simulink library "gmt_Simulink_R2023a"  (R2023a)
settings: Solver=VariableStepAuto  StartTime=0.0  StopTime=10.0  RelTol=1e-3
undefined symbols (not defined in the file or in its folder): MainTank
settings Model: Creator=caksland  LastModifiedBy=jmp8430
settings OptimizationCC: ReuseModelBlockBuffer=off
settings ConfigComp: CovBoundaryAbsTol=1.0e-5

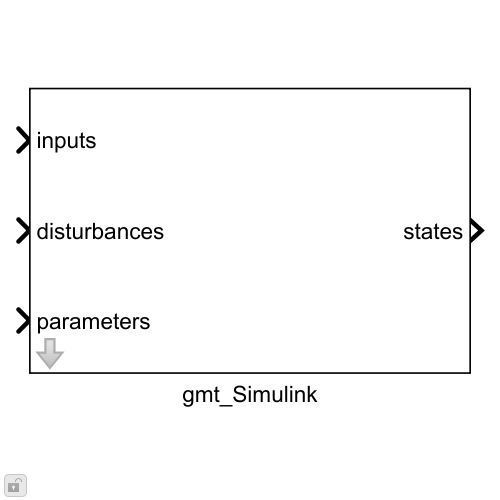
[thumbnail: Simulink's stored preview of the top-level diagram]
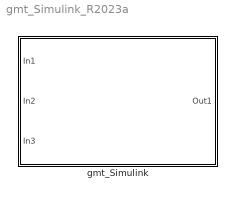
== system gmt_Simulink_R2023a ==
  gmt_Simulink : Subsystem  mask{mdlName=MainTank, x0=[300;300;300;300;6000;300;1500;300], x0_workspace_flg=off}
      mask prompts: mdlName "Model Name (must be object in working directory)"; x0 "Initial State (2):"; x0_workspace_flg "Pull initial conditions from workspace object?"
      settings: CopyFcn=set_param(gcb, 'LinkStatus', 'none');
      mask Callback mdlName:
      | try
      |         blkPath = gcb;
      |         maskObj = Simulink.Mask.get(blkPath);
      |         maskWorkspace = maskObj.getWorkspace();
      |         parameterObj = maskObj.getParameter('mdlName');
      | 
      |         disp('mdlName update callback triggered');
      |         graphObj_name = parameterObj.Value;
      | 
      |         %% Verify variable is in MATLAB workspace (base)
      |         inMATLABworkspace = evalin('base', ['exist(''', graphObj_name, ''', ''var'')']);
      |         assert(inMATLABworkspace,"Variable selected not in MATLAB workspace")
      | 
      |         %% Create graph object variable and verify object is gmt_Graph class
      |         graphObj = evalin('base', graphObj_name);
      |         isGraphObj = isa(graphObj,"gmt_Graph");
      |         assert(isGraphObj,"Variable selected is not a gmt_Graph class")
      | 
      |         %% Grab Basic Graph Object Properties
      |         Nx = graphObj.Properties.Ns;
      |         Ny = graphObj.Properties.Ny;
      |         Nd = graphObj.Properties.Nd;
      |         Nu = graphObj.Properties.Nu;
      |         opt_idx = [graphObj.ModelParameters.Optimization] == true;
      |         Nopt = sum(opt_idx);
      | 
      |         %% Create Mask Prompts
      |         State_Prompt = vertcat(graphObj.States' + ": " + [graphObj.Vertices(graphObj.Properties.Ns_idx).VertexName]');
      |         Output_Prompt = vertcat(graphObj.Outputs);
      |         Input_Prompt = vertcat(graphObj.Inputs' + ": " + [graphObj.InputData.Parent]' + " " + [graphObj.InputData.Description]');
      |         Disturbance_Prompt = vertcat(graphObj.Disturbances' + ": " + [graphObj.Vertices(graphObj.Properties.Nd_idx).VertexName]');
      |         Parameter_Prompt = vertcat([graphObj.ModelParameters(opt_idx).Variable]'+ ": " + [graphObj.ModelParameters(opt_idx).Description]');
      |         CurrentModel_Prompt = "Current Model Loaded: " + parameterObj.Value;
      |         InitialCondition_Prompt = "Initial State (" + string(Nx) + "):";
      | 
      |         %% Update States Info
      |         tbObj = maskObj.getDialogControl("States");
      |         prompt_tmp = State_Prompt;
      | 
      |         if ~isempty(prompt_tmp)
      |             if length(prompt_tmp) > 1
      |                 % set the Prompt value
      |                 tbObj.Prompt = strjoin(convertStringsToChars(prompt_tmp),newline);
      |             else
      |                 tbObj.Prompt = prompt_tmp;
      |             end
      |         else
      |             % set the Prompt value
      |             tbObj.Prompt = "";
      |         end
      | 
      |         %% Update Inputs Info
      |         tbObj = maskObj.getDialogControl("Inputs");
      |         prompt_tmp = Input_Prompt;
      | 
      |         if ~isempty(prompt_tmp)
      |             if length(prompt_tmp) > 1
      |                 % set the Prompt value
      |                 tbObj.Prompt = strjoin(convertStringsToChars(prompt_tmp),newline);
      |             else
      |                 tbObj.Prompt = prompt_tmp;
      |             end
      |         else
      |             % set the Prompt value
      |             tbObj.Prompt = "";
      |         end
      | 
      |         %% Update Outputs Info
      |         tbObj = maskObj.getDialogControl("Outputs");
      |         prompt_tmp = Output_Prompt;
      | 
      |         if ~isempty(prompt_tmp)
      |             if length(prompt_tmp) > 1
      |                 % set the Prompt value
      |                 tbObj.Prompt = strjoin(convertStringsToChars(prompt_tmp),newline);
      |             else
      |                 tbObj.Prompt = prompt_tmp;
      |             end
      |         else
      |             % set the Prompt value
      |             tbObj.Prompt = "";
      |         end
      | 
      |         %% Update Parameters Info
      |         tbObj = maskObj.getDialogControl("Parameters");
      |         prompt_tmp = Parameter_Prompt;
      | 
      |         if ~isempty(prompt_tmp)
      |             if length(prompt_tmp) > 1
      |                 % set the Prompt value
      |                 tbObj.Prompt = strjoin(convertStringsToChars(prompt_tmp),newline);
      |             else
      |                 tbObj.Prompt = prompt_tmp;
      |             end
      |         else
      |             % set the Prompt value
      |             tbObj.Prompt = "";
      |         end
      | 
      |         %% Update Disturbances Info
      |         tbObj = maskObj.getDialogControl("Disturbances");
      |         prompt_tmp = Disturbance_Prompt;
      | 
      |         if ~isempty(prompt_tmp)
      |             if length(prompt_tmp) > 1
      |                 % set the Prompt value
      |                 tbObj.Prompt = strjoin(convertStringsToChars(prompt_tmp),newline);
      |             else
      |                 tbObj.Prompt = prompt_tmp;
      |             end
      |         else
      |             % set the Prompt value
      |             tbObj.Prompt = "";
      |         end
      | 
      |         %% Update mdlName_current Info
      |         tbObj = maskObj.getDialogControl("mdlName_current");
      |         prompt_tmp = CurrentModel_Prompt;
      | 
      |         if ~isempty(prompt_tmp)
      |             if length(prompt_tmp) > 1
      |                 % set the Prompt value
      |                 tbObj.Prompt = strjoin(convertStringsToChars(prompt_tmp),newline);
      |             else
      |                 tbObj.Prompt = prompt_tmp;
      |             end
      |         else
      |             % set the Prompt value
      |             tbObj.Prompt = "";
      |         end
      | 
      |         %% Update Initial Condition Number
      |         tbObj = maskObj.getParameter('x0');
      |         tbObj.Prompt = "Initial State (" + string(Nx) + "):";
      | 
      |         %% Add Initial Conditions
      |         paramObj = maskObj.getParameter('x0_workspace_flg');
      |         rawValue = paramObj.Value;
      |         if strcmp(string(rawValue),"on")
      |             tbObj = maskObj.getParameter('x0');
      |             initCon_values = graphObj.InitialConditions;
      |             %assert(initCon_values,"No initial conditions specified in model")
      |             initCon_str = "[" + strjoin(string(initCon_values),";") + "]";
      |             tbObj.Value = initCon_str;
      |         end
      | 
      |         disp("Updated mask with model info")
      | 
      |          %% Update MATLAB Function Code
      |         blkPath = gcb;
      |         rt = sfroot;
      |         funcBlk = rt.find('-isa', 'Stateflow.EMChart', '-and', 'Path', [blkPath '/MATLAB Function']);
      | 
      |         %% MATLAB Function Prefix
      | 
      |         % Grab State Variable Names
      |         StateVars = graphObj.States';
      |         % Grab Boundary Condition Variable Names
      |         ExtAlgVars = graphObj.Disturbances';
      |         % Grab Control Input Variable Names
      |         InputVars = graphObj.Inputs';
      |         % System Input Packager
      |         funcInput_list = [StateVars; InputVars; ExtAlgVars];
      |         sysfun_mfile_prefix = "";
      |         for i = 1:length(funcInput_list)
      |             sysfun_mfile_prefix(i,1) = funcInput_list(i) + " = u(" + i + ");";
      |         end
      |         %% MATLAB Function Parameters
      |         sysfun_mfile_param = graphObj.ModelMetadata.mfileCode_param;
      |         %% MATLAB Function Body
      |         stateVars_der = StateVars + "_dot";
      |         sysfun_mfile_body = stateVars_der + " = " +  string(graphObj.SystemEquations.RHS) + ";";
      |         %% MATLAB Function Suffix
      |         sysfun_mfile_suffix = "y = [" + strjoin(stateVars_der',";") + "];";
      |         sysfun_mfile_suffix = [sysfun_mfile_suffix; "end"];
      |         %% Create newCode
      |         newCode_str = [sysfun_mfile_prefix;sysfun_mfile_param;sysfun_mfile_body;sysfun_mfile_suffix];
      |         newCode = strjoin(newCode_str,'\n');
      |         funcBlk.Script = newCode;
      | 
      |         %% Update Port Dimensions
      |         totInputs = Nx + Nd + Nu + Nopt;
      |         totOutputs = Nx;
      | 
      |         disp(string(totOutputs))
      |         funcBlk.Inputs.Props.Array.isDynamic = true;
      |         funcBlk.Inputs.Props.Array.Size = "[" + string(totInputs) + " " + string(1) + "]";
      |         funcBlk.Outputs.Props.Array.isDynamic = true;
      |         if totOutputs > 1
      |             funcBlk.Outputs.Props.Array.Size = "[" + string(totOutputs) + " " + string(1) + "]";
      |         else
      |             funcBlk.Outputs.Props.Array.Size =  string(1);
      |         end
      |             disp(funcBlk.Inputs.Props.Array)
      |         disp(funcBlk.Outputs.Props.Array)
      | 
      |         %% Update Mux Dimensions
      |         muxPath = [blkPath '/Mux'];
      |         muxHdl  = get_param(muxPath, 'Handle');
      |         muxPortHdl = get_param(muxPath, 'PortHandles');
      | 
      | 
      |         % Break All Input Lines Into Mux
      |         for k = 1:length(muxPortHdl.Inport)
      |         line = get_param(muxPortHdl.Inport(k), 'Line');
      |             if line ~= -1   % -1 means no line connected
      |                 delete_line(line);
      |             end
      |         end
      | 
      |         % Find and Delete all Terminators
      |         %terms = find_system(blkPath, 'BlockType', 'Terminator', 'LookUnderMasks','all', 'FollowLinks','on');
      | 
      |         %for k = 1:length(terms)
      |         %    delete_block(terms{k});
      |         %end
      | 
      |         % Compute Mux Dimensions
      |         muxNum = 1;
      |         if Nd > 0
      |             muxNum = muxNum + 1;
      |         end
      | 
      |         if Nu > 0
      |             muxNum = muxNum + 1;
      |         end
      | 
      |         if Nopt > 0
      |             muxNum = muxNum + 1;
      |         end
      | 
      |         set_param(muxHdl, 'Inputs', string(muxNum));   % set to 3 inputs
      | 
      |         % Connect Integrator
      |         integratorPath = [blkPath '/Integrator'];
      |         integratorHdl  = get_param(integratorPath, 'Handle');
      |         integratorPortHdl = get_param(integratorPath, 'PortHandles');
      |         add_line(blkPath, integratorPortHdl.Outport(1), muxPortHdl.Inport(1), 'autorouting','on');
      |         PortNum = 1;
      | 
      |         % Connect In1
      |         if Nu > 0
      |             PortNum = PortNum + 1;
      |             In1Path = [blkPath '/In1'];
      |             In1Hdl  = get_param(In1Path, 'Handle');
      |             In1PortHdl = get_param(In1Path, 'PortHandles');
      |             add_line(blkPath, In1PortHdl.Outport(1), muxPortHdl.Inport(PortNum), 'autorouting','on');
      |         else
      | 
      |         end
      | 
      |         % Connect In2
      |         if Nd > 0
      |             PortNum = PortNum + 1;
      |             In2Path = [blkPath '/In2'];
      |             In2Hdl  = get_param(In2Path, 'Handle');
      |             In2PortHdl = get_param(In2Path, 'PortHandles');
      |             add_line(blkPath, In2PortHdl.Outport(1), muxPortHdl.Inport(PortNum), 'autorouting','on');
      |         end
      | 
      |         % Connect In3
      |         if Nopt > 0
      |             PortNum = PortNum + 1;
      |             In3Path = [blkPath '/In3'];
      |             In3Hdl  = get_param(In3Path, 'Handle');
      |             In3PortHdl = get_param(In3Path, 'PortHandles');
      |             add_line(blkPath, In3PortHdl.Outport(1), muxPortHdl.Inport(PortNum), 'autorouting','on');
      |         end
      | 
      |     catch ME
      |         disp(getReport(ME, 'extended'))
      |         rethrow(ME)  % still show Simulink error dialog
      |     end
      mask DialogControl Container7 Prompt: Description
      mask DialogControl Control6 Prompt: This Simulink block can be used to load and simulate a graph model generated with the graph modeling toolbox. The model name must be a gmt_Graph class or subclass object in the MATLAB  workspace. The initial conditions must be a column vector with the same number of rows as there are states.
      mask DialogControl DescGroupVar Prompt: States
      mask DialogControl States Prompt:
      | x1: MainTank: Temperature
      | x2: MainTank: Mass
      mask DialogControl Container3 Prompt: Outputs
      mask DialogControl Container4 Prompt: Inputs
      mask DialogControl Inputs Prompt:
      | u1: MainTank Inlet Mass Flow 1
      | u2: MainTank Outlet Mass Flow 1
      mask DialogControl Container5 Prompt: Disturbances
      mask DialogControl Disturbances Prompt: x4: MainTank: Source Temperature
      mask DialogControl Container6 Prompt: Parameters
      mask DialogControl ParameterGroupVar Prompt: Model Configuration
      mask DialogControl mdlName_current Prompt: Current Model Loaded: MainTank
      mask Display:
      | port_label('input', 1, 'inputs');
      | port_label('input', 2, 'disturbances');
      | port_label('input', 3, 'parameters');
      | port_label('output', 1, 'states');

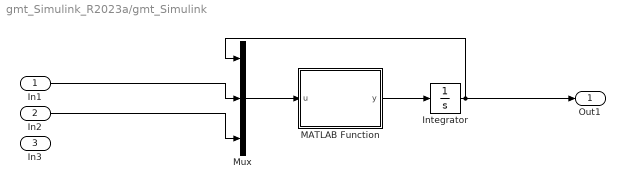
== system gmt_Simulink_R2023a/gmt_Simulink ==
  In1 : Inport
  In2 : Inport  Port=2
  In3 : Inport  Port=3
  Integrator : Integrator  InitialCondition=x0
  MATLAB Function : MATLAB Function  TreatAsAtomicUnit=on
  Mux : Mux  Inputs=3
  Out1 : Outport
  wires:
  MATLAB Function/1(y) -> Integrator/1
  Integrator/1 -> Out1/1, Mux/1
  Mux/1 -> MATLAB Function/1(u)
  In1/1 -> Mux/2
  In2/1 -> Mux/3

== matlab function gmt_Simulink_R2023a/gmt_Simulink/MATLAB Function ==
  data: u input size=[5 1]; y output size=[2 1]
function y = fcn(u)
x1 = u(1);
x2 = u(2);
u1 = u(3);
u2 = u(4);
x4 = u(5);
cp_f = 3300;
Rho = 1090;
V = 0.002;
x1_dot = -(cp_f*u2*x1 - cp_f*u1*x4 + cp_f*x1*(u1 - u2))/(cp_f*x2);
x2_dot = u1 - u2;
y = [x1_dot;x2_dot];
end
